simulink model "Ex7_1"  (R2022b)
settings: Solver=VariableStepAuto  StartTime=0.0  StopTime=0.02  RelTol=1e-3
libraries: instrumentseriallib x2
settings Model: Creator=10043  LastModifiedBy=10043

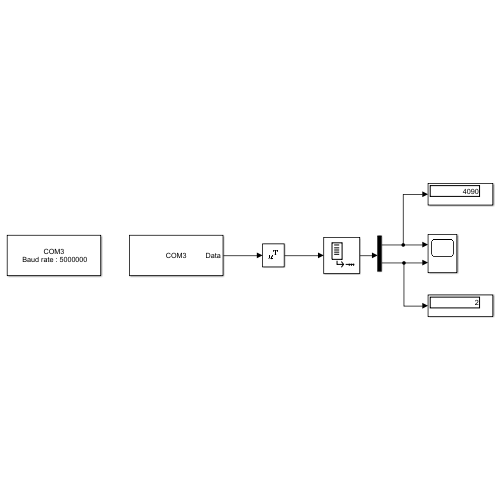
[thumbnail: Simulink's stored preview of the top-level diagram]
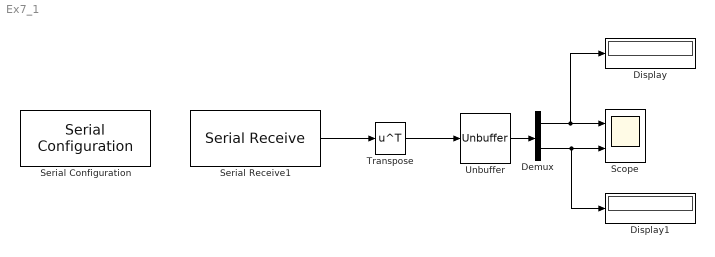
== system Ex7_1 ==
  Demux : Demux  Outputs=2
  Display : Display
  Display1 : Display
  Scope : Scope  NumInputPorts=2
  Serial Configuration : instrumentseriallib/Serial Configuration  Priority=-200000  PortSel=COM3  Port=COM3  ComPort=COM3  BaudRate=5000000  DataBits=8  Parity=none  StopBits=1  ByteOrder=little-endian  FlowControl=none  Timeout=10  SimulateUsing=Interpreted execution  BlockInModel=on  aMode=1
  Serial Receive1 : instrumentseriallib/Serial Receive  Priority=1  PortSel=COM3  Port=COM3  ComPort=COM3  DataType=uint16  SaveDataType=uint8  ToggleHeader=on  Header=[0x53 0x53]  ToggleTerminator=on  Terminator=Custom terminator  CustomTerminator=[0x45 0x45]  InputFormat=Column major  ToggleDataSize=on  DataSize=[2 16]  EnableBlockingMode=on  ActionDataUnavailable=Output last received value  ActionWhenDataUnavailable=Output last received value  CustomValue=0  SampleTime=1e-5  SimulateUsing=Interpreted execution  BlockInModel=on  aMode=1
  Transpose : Math  Operator=transpose
  Unbuffer : Unbuffer
  wires:
  Demux/2 -> Display1/1, Scope/2
  Serial Receive1/1 -> Transpose/1
  Transpose/1 -> Unbuffer/1
  Unbuffer/1 -> Demux/1
  Demux/1 -> Display/1, Scope/1
